simulink model "Pendulum_block"  (R2015a)
settings: Solver=ode45  StartTime=0.0  StopTime=20.0  RelTol=1e-3
settings Model: ExtModeTrigMode=oneshot  ExtModeArmWhenConnect=off  Creator=PC  LastModifiedBy=Alessandra
settings DataIOCC: LimitDataPoints=off  SignalLoggingSaveFormat=ModelDataLogs
settings OptimizationCC: BlockReduction=off  BooleanDataType=off  ExpressionDepthLimit=2147483647  InitFltsAndDblsToZero=on
settings DebuggingCC: SaveWithParameterizedLinksMsg=none  UnderspecifiedInitializationDetection=Classic  MergeDetectMultiDrivingBlocksExec=none  SignalResolutionControl=TryResolveAllWithWarning  MultiTaskDSMMsg=warning  MultiTaskCondExecSysMsg=none  FcnCallInpInsideContextMsg=UseLocalSettings  StateNameClashWarn=warning
settings HardwareCC: TargetUnknown=on
settings GRTTargetCC: TargetFcnLib=ansi_tfl_tmw.mat  CombineOutputUpdateFcns=off  GRTInterface=on

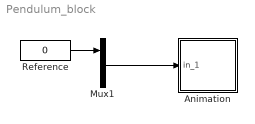
== system Pendulum_block ==
  Animation : Subsystem  mask(Pendulum plot){RefBlock=Reference}
      mask prompts: RefBlock "DC reference signal block name:"
      mask help: Pendulum plot
      mask Help: Pendulum animation function using Handle graphics.
      mask Display: plot([-10 10],[0 0],[-2 -2 2 2],[0 1 1 0],[0 3],[1 5])
  Mux1 : Mux  Inputs=2
  Reference : Constant  Value=0
  wires:
  Mux1/1 -> Animation/1(in_1)
  Reference/1 -> Mux1/1

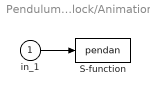
== system Pendulum_block/Animation ==
  in_1 : Inport
  S-function : S-Function  FunctionName=pendan  Parameters=RefBlock
      settings: DeleteFcn=pendan([],[],[],'DeleteBlock');
  wires:
  in_1/1 -> S-function/1
